simulink model "quad_3_ref_NN"  (R2018b)
settings: Solver=VariableStepAuto  StartTime=0.0  StopTime=20  RelTol=1e-3
undefined symbols (not defined in the file or in its folder): options
libraries: neural x70, simulink x3
(part 4 of 4)

== system quad_3_ref_NN/nn_1/Layer 3/Delays 1 ==
  "p{3}" : Inport  PortDimensions=30
      mask Display: e = 0.06;c1 = [120 230 180]/255;c2 = ([120 230 180]+0)/(256+128);c3 = ([120 230 180]+128)/(256+128);patch([0 1 1 0],[0 0 1 1],c1);patch([0 1 1 1-e 1-e 0+e],[0 0 1 1-e 0+e 0+e],c2);patch([0 0 1 1-e 0+e 0+e],[0 1 1 1-e 1-e 0+e],c3);plot([0 1 1 0 0],[0 0 1 1 0]);
  mux : Mux  Inputs=1
      mask Display: e = 0.06;c1 = [120 150 230]/255;c2 = ([120 150 230]+0)/383;c3 = ([120 150 230]+128)/383;patch([0 1 1 0],[0 0 1 1],c1);patch([0 1 1 1-e 1-e 0+e],[0 0 1 1-e 0+e 0+e],c2);patch([0 0 1 1-e 0+e 0+e],[0 1 1 1-e 1-e 0+e],c3);plot([0 1 1 0 0],[0 0 1 1 0]);disp('Mux')
  "pd{3,2}" : Outport
      mask Display: e = 0.06;c1 = [120 230 180]/255;c2 = ([120 230 180]+0)/(256+128);c3 = ([120 230 180]+128)/(256+128);patch([0 1 1 0],[0 0 1 1],c1);patch([0 1 1 1-e 1-e 0+e],[0 0 1 1-e 0+e 0+e],c2);patch([0 0 1 1-e 0+e 0+e],[0 1 1 1-e 1-e 0+e],c3);plot([0 1 1 0 0],[0 0 1 1 0]);
  wires:
  "p{3}"/1 -> mux/1
  mux/1 -> "pd{3,2}"/1

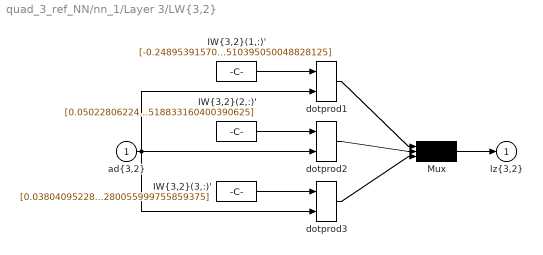
== system quad_3_ref_NN/nn_1/Layer 3/LW{3,2} ==
  "ad{3,2}" : Inport  PortDimensions=30
      mask Display: e = 0.06;c1 = [120 230 180]/255;c2 = ([120 230 180]+0)/(256+128);c3 = ([120 230 180]+128)/(256+128);patch([0 1 1 0],[0 0 1 1],c1);patch([0 1 1 1-e 1-e 0+e],[0 0 1 1-e 0+e 0+e],c2);patch([0 0 1 1-e 0+e 0+e],[0 1 1 1-e 1-e 0+e],c3);plot([0 1 1 0 0],[0 0 1 1 0]);
  "IW{3,2}(1,:)'" : Constant  Value=[-0.248953915706701278676149513557902537286281585693359375;0.2371431390955625329031164483239990659058094024658203125;0.022510892670564323914117466074458207003772258758544921875;-0.1695964430487302276873151640756987035274505615234375;0.2662051507641287617644820784335024654865264892578125;0.159738407958096129135583396418951451778411865234375;-0.069179901092365270187656278721988201141357421875;-0.2415885267418215465173858547132113017141819000244140625;0.2074725232813476039073208312402130104601383209228515625;0.26555184106539841959460090947686694562435150146484375;-0.414383550795543398326259421082795597612857818603515625;-0.03651746886232942745920126981218345463275909423828125;-0.12131449747704127484215774757103645242750644683837890625;-0.288193640410273788088346691438346169888973236083984375;-0.31423996458324332525791078296606428921222686767578125;0.350468194191082715871488062475691549479961395263671875;0.307568601719888923273771297317580319941043853759765625;-0.380853374671231481585209621698595583438873291015625;-0.00333715397267724152297052597759829950518906116485595703125;0.3201379362005523088186009772471152245998382568359375;-0.2511782717737440773220214396133087575435638427734375;0.1145372947914090333565440005259006284177303314208984375;0.255821682431940977675566273319418542087078094482421875;-0.1738936712714936050350189589153160341084003448486328125;-0.13794698641003766415025211244937963783740997314453125;-0.3530252178733721546421975290286354720592498779296875;-0.260489773985550954193968209438025951385498046875;-0.01079630895070284209158462118693933007307350635528564453125;-0.1518295694095441461524131909754942171275615692138671875;0.1836876092094939239007800324543495662510395050048828125]
      mask Display: e = 0.06;c1 = [120 150 230]/255;c2 = ([120 150 230]+0)/383;c3 = ([120 150 230]+128)/383;patch([0 1 1 0],[0 0 1 1],c1);patch([0 1 1 1-e 1-e 0+e],[0 0 1 1-e 0+e 0+e],c2);patch([0 0 1 1-e 0+e 0+e],[0 1 1 1-e 1-e 0+e],c3);plot([0 1 1 0 0],[0 0 1 1 0]);disp('weights');
  "IW{3,2}(2,:)'" : Constant  Value=[0.050228062243247661999845377067686058580875396728515625;-0.035752645029441219859389633484170190058648586273193359375;0.027530532749164289552101791969107580371201038360595703125;-0.01543245227947603707974177922324088285677134990692138671875;0.0087180679113108595912340348377256304956972599029541015625;0.003818980617202629747330977494357284740544855594635009765625;0.030875403824292262100481565312293241731822490692138671875;-0.00449058897316372516994587016370132914744317531585693359375;0.0235664784172817769192231907027235138230025768280029296875;-0.030042127931204538893172895086536300368607044219970703125;0.0169147844369839338296568342911996296606957912445068359375;0.003491503281852189992384705163885882939212024211883544921875;0.0148000691151590514638147766390829929150640964508056640625;0.0120305261847679957620815827112892293371260166168212890625;0.035075392682133783861520015534551930613815784454345703125;0.01400946722449833252432949137755713309161365032196044921875;-0.02857377395372150130636867970679304562509059906005859375;0.0249754584312845105686928803834234713576734066009521484375;-0.022336894082788126547622908901757909916341304779052734375;-0.0167703692824410499628839943397906608879566192626953125;0.0088604466339316685641325221922670607455074787139892578125;-0.005428789579366931870862966746926758787594735622406005859375;-0.0235670001636054428362232471272363909520208835601806640625;0.01716801641922127696915367778274230659008026123046875;-0.037760267955889957602888529208939871750771999359130859375;0.0376112459169738733155696763788000680506229400634765625;0.002710204679426350161952630202222280786372721195220947265625;-0.0125966260913606999116698403895497904159128665924072265625;-0.01822272848687704616121862954969401471316814422607421875;-0.02138659124138354850064303036560886539518833160400390625]
      mask Display: e = 0.06;c1 = [120 150 230]/255;c2 = ([120 150 230]+0)/383;c3 = ([120 150 230]+128)/383;patch([0 1 1 0],[0 0 1 1],c1);patch([0 1 1 1-e 1-e 0+e],[0 0 1 1-e 0+e 0+e],c2);patch([0 0 1 1-e 0+e 0+e],[0 1 1 1-e 1-e 0+e],c3);plot([0 1 1 0 0],[0 0 1 1 0]);disp('weights');
  "IW{3,2}(3,:)'" : Constant  Value=[0.038040952289257239093966944665226037614047527313232421875;-0.03287470104792077074673528613857342861592769622802734375;0.0249384610736344269898978609489859081804752349853515625;-0.004896497330191327927717548362807065132074058055877685546875;0.00054051835928161577442263574511116530629806220531463623046875;0.00480313973110746243733171212397792260162532329559326171875;0.0092603418604377540912508948167669586837291717529296875;-0.0024756602082472538295387920470602693967521190643310546875;0.035473773570854072456626226994558237493038177490234375;-0.0294771906179413477333550730463684885762631893157958984375;0.0139583565886113591947292889017262496054172515869140625;-0.0083130164261612481124696927281547687016427516937255859375;0.006849797305116592065210578965661625261418521404266357421875;-0.00240469885496467049301738683197982027195394039154052734375;0.029444019242555706517006086642140871845185756683349609375;-0.00442716887063401669244466773989188368432223796844482421875;-0.02331963847812172641038586107242736034095287322998046875;0.00875901422854506901682913877493774634785950183868408203125;-0.0086328667142883085128257647511418326757848262786865234375;6.022995479666552742781249207837390713393688201904296875e-05;0.007123150480693015741684437358571813092567026615142822265625;-0.00130636627904807435529566106424681493081152439117431640625;-0.005252187332847592544926573765451394137926399707794189453125;0.0243212768199290996218309146570391021668910980224609375;-0.03127476605162103628909875396857387386262416839599609375;0.031806604782959942145925680279106018133461475372314453125;-0.00709297547331089010824722862480484764091670513153076171875;-0.0252802882746179964634780645837963675148785114288330078125;-0.03068706696818331025600201655834098346531391143798828125;-0.028535215154707527229760444242856465280055999755859375]
      mask Display: e = 0.06;c1 = [120 150 230]/255;c2 = ([120 150 230]+0)/383;c3 = ([120 150 230]+128)/383;patch([0 1 1 0],[0 0 1 1],c1);patch([0 1 1 1-e 1-e 0+e],[0 0 1 1-e 0+e 0+e],c2);patch([0 0 1 1-e 0+e 0+e],[0 1 1 1-e 1-e 0+e],c3);plot([0 1 1 0 0],[0 0 1 1 0]);disp('weights');
  Mux : Mux  Inputs=3
      mask Display: e = 0.06;c1 = [120 150 230]/255;c2 = ([120 150 230]+0)/383;c3 = ([120 150 230]+128)/383;patch([0 1 1 0],[0 0 1 1],c1);patch([0 1 1 1-e 1-e 0+e],[0 0 1 1-e 0+e 0+e],c2);patch([0 0 1 1-e 0+e 0+e],[0 1 1 1-e 1-e 0+e],c3);plot([0 1 1 0 0],[0 0 1 1 0]);disp('Mux');
  dotprod1 : neural/Weight Functions/dotprod
  dotprod2 : neural/Weight Functions/dotprod
  dotprod3 : neural/Weight Functions/dotprod
  "lz{3,2}" : Outport
      mask Display: e = 0.06;c1 = [120 230 180]/255;c2 = ([120 230 180]+0)/(256+128);c3 = ([120 230 180]+128)/(256+128);patch([0 1 1 0],[0 0 1 1],c1);patch([0 1 1 1-e 1-e 0+e],[0 0 1 1-e 0+e 0+e],c2);patch([0 0 1 1-e 0+e 0+e],[0 1 1 1-e 1-e 0+e],c3);plot([0 1 1 0 0],[0 0 1 1 0]);
  wires:
  "IW{3,2}(1,:)'"/1 -> dotprod1/1
  "ad{3,2}"/1 -> dotprod1/2, dotprod2/2, dotprod3/2
  dotprod1/1 -> Mux/1
  "IW{3,2}(2,:)'"/1 -> dotprod2/1
  dotprod2/1 -> Mux/2
  "IW{3,2}(3,:)'"/1 -> dotprod3/1
  dotprod3/1 -> Mux/3
  Mux/1 -> "lz{3,2}"/1

== matlab function quad_3_ref_NN/MATLAB Function ==
  data: r1 input; F output; r2 input; r3 input; x3 input; x6 input; x7 input; x8 input; x10 input; x11 input; tau_phi output; tau_theta output; tau_psi output
function [F,tau_phi,tau_theta,tau_psi] = fcn(r1,r2,r3,x3,x6,x7,x8,x10,x11)
%initialization
m=1.4;
g=9.81;
F= m*g-10*(x3-r1)+3*x6;
tau_phi=-(x7-r2)-x10;
tau_theta=-(x8-r3)-x11;
tau_psi=0;
